simulink model "MPC_MG secondary"  (R2021b)
settings: Solver=ode23tb  StartTime=0.0  StopTime=5  RelTol=1e-3
model workspace (MAT data in the model file):
  Ts : Simulink.Parameter (value not decoded)
  secondary_on : Simulink.Parameter (value not decoded)
values from neighbouring files (symbols this model uses):
  a12 = 0    [Four_DG_MG_PrimaryOnlyScript.m]    (also in MPC_MG_script_raw_dmpc.m; MPC_MG_secondary_script.m)
  a14 = 0    [Four_DG_MG_PrimaryOnlyScript.m]    (also in MPC_MG_script_raw_dmpc.m; MPC_MG_secondary_script.m)
  a21 = 1    [Four_DG_MG_PrimaryOnlyScript.m]    (also in MPC_MG_script_raw_dmpc.m; MPC_MG_secondary_script.m)
  a23 = 0    [Four_DG_MG_PrimaryOnlyScript.m]    (also in MPC_MG_script_raw_dmpc.m; MPC_MG_secondary_script.m)
  a32 = 1    [Four_DG_MG_PrimaryOnlyScript.m]    (also in MPC_MG_script_raw_dmpc.m; MPC_MG_secondary_script.m)
  a34 = 0    [Four_DG_MG_PrimaryOnlyScript.m]    (also in MPC_MG_script_raw_dmpc.m; MPC_MG_secondary_script.m)
  a41 = 1    [Four_DG_MG_PrimaryOnlyScript.m]    (also in MPC_MG_script_raw_dmpc.m; MPC_MG_secondary_script.m)
  a43 = 0    [Four_DG_MG_PrimaryOnlyScript.m]    (also in MPC_MG_script_raw_dmpc.m; MPC_MG_secondary_script.m)
  b1v = 1    [Four_DG_MG_PrimaryOnlyScript.m]    (also in MPC_MG_script_raw_dmpc.m; MPC_MG_secondary_script.m; MPG_MG_July.m; MPG_MG_freq_script.m)
  b1w = 1    [Four_DG_MG_PrimaryOnlyScript.m]    (also in MPC_MG_script_raw_dmpc.m; MPC_MG_secondary_script.m; MPG_MG_July.m; MPG_MG_freq_script.m)
  b2v = 0    [Four_DG_MG_PrimaryOnlyScript.m]    (also in MPC_MG_script_raw_dmpc.m; MPC_MG_secondary_script.m; MPG_MG_July.m; MPG_MG_freq_script.m)
  b2w = 0    [Four_DG_MG_PrimaryOnlyScript.m]    (also in MPC_MG_script_raw_dmpc.m; MPC_MG_secondary_script.m; MPG_MG_July.m; MPG_MG_freq_script.m)
  b3v = 0    [Four_DG_MG_PrimaryOnlyScript.m]    (also in MPC_MG_script_raw_dmpc.m; MPC_MG_secondary_script.m; MPG_MG_July.m; MPG_MG_freq_script.m)
  b3w = 0    [Four_DG_MG_PrimaryOnlyScript.m]    (also in MPC_MG_script_raw_dmpc.m; MPC_MG_secondary_script.m; MPG_MG_July.m; MPG_MG_freq_script.m)
  b4v = 0    [Four_DG_MG_PrimaryOnlyScript.m]    (also in MPC_MG_script_raw_dmpc.m; MPC_MG_secondary_script.m; MPG_MG_July.m; MPG_MG_freq_script.m)
  b4w = 0    [Four_DG_MG_PrimaryOnlyScript.m]    (also in MPC_MG_script_raw_dmpc.m; MPC_MG_secondary_script.m; MPG_MG_July.m; MPG_MG_freq_script.m)
  C_f = 50e-6    (= 5e-05)    [Four_DG_MG_PrimaryOnlyScript.m]    (also in MPC_MG_script.m; MPC_MG_script_raw_dmpc.m; MPC_MG_secondary_script.m; MPG_MG_July.m)
  cf = 60    [Four_DG_MG_PrimaryOnlyScript.m]    (also in MPC_MG_script_raw_dmpc.m = 40; MPC_MG_secondary_script.m = 40; MPG_MG_July.m = 100; MPG_MG_freq_script.m = 100)
  cv = 60    [Four_DG_MG_PrimaryOnlyScript.m]    (also in MPC_MG_script_raw_dmpc.m = 40; MPC_MG_secondary_script.m = 40; MPG_MG_July.m = 100; MPG_MG_freq_script.m = 100)
  f_c = 5000    [Four_DG_MG_PrimaryOnlyScript.m]    (also in MPC_MG_script.m = 40000; MPC_MG_script_raw_dmpc.m = 40000; MPC_MG_secondary_script.m = 40000; MPG_MG_July.m = 50000)
  kL = 1e-5    (= 1e-05)    [Four_DG_MG_PrimaryOnlyScript.m]    (also in MPC_MG_script.m = 1e-08; MPC_MG_script_raw_dmpc.m = 1e-08; MPC_MG_secondary_script.m = 1e-07; MPG_MG_July.m = 1e-07)
  L_f = 1.35e-3    (= 0.00135)    [Four_DG_MG_PrimaryOnlyScript.m]    (also in MPC_MG_script.m; MPC_MG_script_raw_dmpc.m; MPC_MG_secondary_script.m; MPG_MG_July.m)
  L_in1 = 0.35e-3    (= 0.00035)    [Four_DG_MG_PrimaryOnlyScript.m]    (also in MPC_MG_script.m; MPC_MG_script_raw_dmpc.m; MPC_MG_secondary_script.m; MPG_MG_July.m)
  L_in2 = 0.35e-3    (= 0.00035)    [Four_DG_MG_PrimaryOnlyScript.m]    (also in MPC_MG_script.m; MPC_MG_script_raw_dmpc.m; MPC_MG_secondary_script.m; MPG_MG_July.m)
  L_in3 = 0.35e-3    (= 0.00035)    [Four_DG_MG_PrimaryOnlyScript.m]    (also in MPC_MG_script.m; MPC_MG_script_raw_dmpc.m; MPC_MG_secondary_script.m; MPG_MG_July.m)
  L_in4 = 0.35e-3    (= 0.00035)    [Four_DG_MG_PrimaryOnlyScript.m]    (also in MPC_MG_script.m; MPC_MG_script_raw_dmpc.m; MPC_MG_secondary_script.m; MPG_MG_July.m)
  LD_ref1 = 800e-6    (= 0.0008)    [Four_DG_MG_PrimaryOnlyScript.m]    (also in MPC_MG_script.m = 0.0003; MPC_MG_script_raw_dmpc.m = 0.0003; MPC_MG_secondary_script.m = 0.0001; MPG_MG_July.m = 0.0004)
  lo_co = 0.2    [Four_DG_MG_PrimaryOnlyScript.m]    (also in MPC_MG_script.m = 0.05; MPC_MG_script_raw_dmpc.m; MPC_MG_secondary_script.m = 0.08; MPG_MG_July.m = 0.15)
  m_p1 = 9.4e-5/droopDivide    (= 9.4e-05)    [Four_DG_MG_PrimaryOnlyScript.m]    (also in MPC_MG_script.m; MPC_MG_script_raw_dmpc.m; MPC_MG_secondary_script.m; MPG_MG_July.m)
  m_p2 = 9.4e-5/droopDivide    (= 9.4e-05)    [Four_DG_MG_PrimaryOnlyScript.m]    (also in MPC_MG_script.m; MPC_MG_script_raw_dmpc.m; MPC_MG_secondary_script.m; MPG_MG_July.m)
  m_p3 = 12.5e-5/droopDivide    (= 0.000125)    [Four_DG_MG_PrimaryOnlyScript.m]    (also in MPC_MG_script.m; MPC_MG_script_raw_dmpc.m; MPC_MG_secondary_script.m; MPG_MG_July.m)
  m_p4 = 12.5e-5/droopDivide    (= 0.000125)    [Four_DG_MG_PrimaryOnlyScript.m]    (also in MPC_MG_script.m; MPC_MG_script_raw_dmpc.m; MPC_MG_secondary_script.m; MPG_MG_July.m)
  n_q1 = 1.3e-3/droopDivide2    (= 0.00013)    [Four_DG_MG_PrimaryOnlyScript.m]    (also in MPC_MG_script.m; MPC_MG_script_raw_dmpc.m; MPC_MG_secondary_script.m; MPG_MG_July.m)
  n_q2 = 1.3e-3/droopDivide2    (= 0.00013)    [Four_DG_MG_PrimaryOnlyScript.m]    (also in MPC_MG_script.m; MPC_MG_script_raw_dmpc.m; MPC_MG_secondary_script.m; MPG_MG_July.m)
  n_q3 = 1.5e-3/droopDivide2    (= 0.00015)    [Four_DG_MG_PrimaryOnlyScript.m]    (also in MPC_MG_script.m; MPC_MG_script_raw_dmpc.m; MPC_MG_secondary_script.m; MPG_MG_July.m)
  n_q4 = 1.5e-3/droopDivide2    (= 0.00015)    [Four_DG_MG_PrimaryOnlyScript.m]    (also in MPC_MG_script.m; MPC_MG_script_raw_dmpc.m; MPC_MG_secondary_script.m; MPG_MG_July.m)
  R_f = 0.1    [Four_DG_MG_PrimaryOnlyScript.m]    (also in MPC_MG_script.m; MPC_MG_script_raw_dmpc.m; MPC_MG_secondary_script.m; MPG_MG_July.m)
  R_in1 = 0.03    [Four_DG_MG_PrimaryOnlyScript.m]    (also in MPC_MG_script.m; MPC_MG_script_raw_dmpc.m; MPC_MG_secondary_script.m; MPG_MG_July.m)
  R_in2 = 0.03    [Four_DG_MG_PrimaryOnlyScript.m]    (also in MPC_MG_script.m; MPC_MG_script_raw_dmpc.m; MPC_MG_secondary_script.m; MPG_MG_July.m)
  R_in3 = 0.03    [Four_DG_MG_PrimaryOnlyScript.m]    (also in MPC_MG_script.m; MPC_MG_script_raw_dmpc.m; MPC_MG_secondary_script.m; MPG_MG_July.m)
  R_in4 = 0.03    [Four_DG_MG_PrimaryOnlyScript.m]    (also in MPC_MG_script.m; MPC_MG_script_raw_dmpc.m; MPC_MG_secondary_script.m; MPG_MG_July.m)
  time_thresh = 0.6    [Four_DG_MG_PrimaryOnlyScript.m]    (also in MPC_MG_script_raw_dmpc.m = 1.5; MPC_MG_secondary_script.m = 2; MPG_MG_July.m = 0.5; MPG_MG_freq_script.m = 0.5)
  Ts = 10e-6    (= 1e-05)    [Four_DG_MG_PrimaryOnlyScript.m]    (also in MPC_MG_script.m; MPC_MG_script_raw_dmpc.m; MPC_MG_secondary_script.m; MPG_MG_July.m)
  V_nom = 220*sqrt(2)    [Four_DG_MG_PrimaryOnlyScript.m]    (also in MPC_MG_script.m; MPC_MG_script_raw_dmpc.m; MPC_MG_secondary_script.m; MPG_MG_July.m)
  Vdc = 600    [Four_DG_MG_PrimaryOnlyScript.m]    (also in MPC_MG_script.m; MPC_MG_script_raw_dmpc.m; MPC_MG_secondary_script.m; MPG_MG_July.m)
  w_c_high = 2*pi*50    (= 314.159265359)    [Four_DG_MG_PrimaryOnlyScript.m]    (also in MPC_MG_script.m; MPC_MG_script_raw_dmpc.m; MPC_MG_secondary_script.m; MPG_MG_July.m)
  w_nom = 2*pi*50    (= 314.159265359)    [Four_DG_MG_PrimaryOnlyScript.m]    (also in MPC_MG_script.m; MPC_MG_script_raw_dmpc.m; MPC_MG_secondary_script.m; MPG_MG_July.m)
undefined symbols (not defined in the file or in its folder): i
libraries: spsThreePhaseSeriesRLCBranchLib x18, spsThreePhaseVIMeasurementLib x12, spsabctodq0Lib x12, eeGeneralControl x10, dspswit3 x5, powerlib x5, spsPMUPLLBasedPositiveSequenceLib x4, spsDCVoltageSourceLib x4, spsSeriesRLCBranchLib x4, spsTwoLevelConverterLib x4, spsThreePhaseSeriesRLCLoadLib x3, powerlib_meascontrol x3
(part 3 of 3)

== system MPC_MG secondary/Voltage Source Inverter 4/3to2 1 ==
  "Vabc_o " : Inport
  Add : Sum  Inputs=+++
  Constant : Constant  Value=exp(i*2*pi/3)
  Constant1 : Constant  Value=2/3
  Demux : Demux  Outputs=3
  Math Function : Math  Operator=square  SignedPower=on  SaturateOnIntegerOverflow=on
  Product : Product  RndMeth=Zero
  Product1 : Product  RndMeth=Zero
  Product2 : Product  RndMeth=Zero
  Vo : Outport  VectorParamsAs1DForOutWhenUnconnected=off
  wires:
  Add/1 -> Product/1
  Demux/1 -> Add/1
  Constant1/1 -> Product/2
  Product1/1 -> Add/2
  Constant/1 -> Product1/1, Math Function/1
  Demux/2 -> Product1/2
  Math Function/1 -> Product2/1
  Demux/3 -> Product2/2
  Product2/1 -> Add/3
  Product/1 -> Vo/1
  "Vabc_o "/1 -> Demux/1

== system MPC_MG secondary/Voltage Source Inverter 4/3to2 2 ==
  "Iabc_o " : Inport
  Add : Sum  Inputs=+++
  Constant : Constant  Value=exp(i*2*pi/3)
  Constant1 : Constant  Value=2/3
  Demux : Demux  Outputs=3
  Math Function : Math  Operator=square  SignedPower=on  SaturateOnIntegerOverflow=on
  Product : Product  RndMeth=Zero
  Product1 : Product  RndMeth=Zero
  Product2 : Product  RndMeth=Zero
  Il : Outport  VectorParamsAs1DForOutWhenUnconnected=off
  wires:
  Add/1 -> Product/1
  Demux/1 -> Add/1
  Constant1/1 -> Product/2
  Product1/1 -> Add/2
  Constant/1 -> Product1/1, Math Function/1
  Demux/2 -> Product1/2
  Math Function/1 -> Product2/1
  Demux/3 -> Product2/2
  Product2/1 -> Add/3
  Product/1 -> Il/1
  "Iabc_o "/1 -> Demux/1

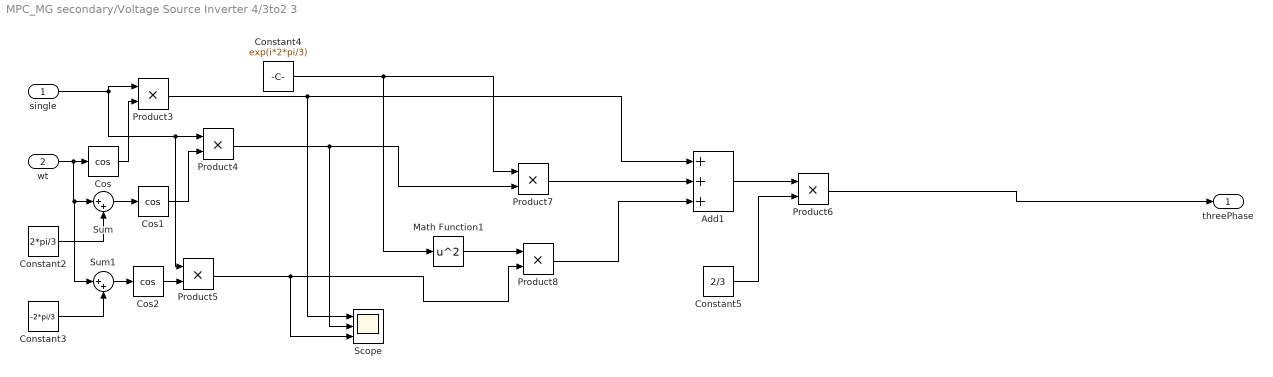
== system MPC_MG secondary/Voltage Source Inverter 4/3to2 3 ==
  "single " : Inport
  "wt " : Inport  Port=2
  Add1 : Sum  Inputs=+++
  Constant2 : Constant  Value=2*pi/3
  Constant3 : Constant  Value=-2*pi/3
  Constant4 : Constant  Value=exp(i*2*pi/3)
  Constant5 : Constant  Value=2/3
  Cos : Trigonometry  Operator=cos
  Cos1 : Trigonometry  Operator=cos
  Cos2 : Trigonometry  Operator=cos
  Math Function1 : Math  Operator=square  SignedPower=on  SaturateOnIntegerOverflow=on
  Product{3..8} (6 alike) : Product  RndMeth=Zero
  Scope : Scope  NumInputPorts=3
  Sum : Sum  Inputs=|++
  Sum1 : Sum  Inputs=|++
  threePhase : Outport  VectorParamsAs1DForOutWhenUnconnected=off
  wires:
  "single "/1 -> Product5/1, Product4/1, Product3/1
  Cos/1 -> Product3/2
  Constant2/1 -> Sum/2
  Sum/1 -> Cos1/1
  Cos1/1 -> Product4/2
  "wt "/1 -> Sum1/1, Sum/1, Cos/1
  Constant3/1 -> Sum1/2
  Sum1/1 -> Cos2/1
  Cos2/1 -> Product5/2
  Constant4/1 -> Product7/1, Math Function1/1
  Product7/1 -> Add1/2
  Add1/1 -> Product6/1
  Product8/1 -> Add1/3
  Product5/1 -> Scope/3, Product8/2
  Product6/1 -> threePhase/1
  Product3/1 -> Scope/1, Add1/1
  Constant5/1 -> Product6/2
  Product4/1 -> Scope/2, Product7/2
  Math Function1/1 -> Product8/1

== system MPC_MG secondary/Voltage Source Inverter 4/Droop for secondary control2 ==
  P : Inport
  w_nom : Inport  Port=2
  V_nom : Inport  Port=3
  Q : Inport  Port=4
  Gain4 : Gain  Gain=n_q
  Gain5 : Gain  Gain=m_p
  Integrator : Integrator  WrapState=on  WrappedStateUpperValue=2*pi  WrappedStateLowerValue=0
  Sum1 : Sum  Inputs=|+-
  Sum2 : Sum  Inputs=|+-
  Vref : Outport
  wt : Outport  Port=2
  wo : Outport  Port=3
  wires:
  P/1 -> Gain5/1
  w_nom/1 -> Sum2/1
  Gain5/1 -> Sum2/2
  Sum2/1 -> wo/1, Integrator/1  "w"
  Integrator/1 -> wt/1
  V_nom/1 -> Sum1/1  "Vod_s"
  Gain4/1 -> Sum1/2
  Q/1 -> Gain4/1
  Sum1/1 -> Vref/1  "Vod_s"

== system MPC_MG secondary/Voltage Source Inverter 4/Low-pass filter ==
  p_hat : Inport
  q_hat : Inport  Port=2
  Low-Pass Filter (Discrete or Continuous) : eeGeneralControl/Low-Pass Filter (Discrete or Continuous)  K=1  T=lo_co  B=inf  A=-inf  init_option=Inherited from block input  x0=0  Ts=-1
  Low-Pass Filter (Discrete or Continuous)1 : eeGeneralControl/Low-Pass Filter (Discrete or Continuous)  K=1  T=lo_co  B=inf  A=-inf  init_option=Inherited from block input  x0=0  Ts=-1
  P : Outport
  Q : Outport  Port=2
  wires:
  q_hat/1 -> Low-Pass Filter (Discrete or Continuous)1/1
  Low-Pass Filter (Discrete or Continuous)1/1 -> Q/1  "Q"
  Low-Pass Filter (Discrete or Continuous)/1 -> P/1  "P"
  p_hat/1 -> Low-Pass Filter (Discrete or Continuous)/1

== system MPC_MG secondary/Voltage Source Inverter 4/PQ calculator ==
  Vod : Inport
  Voq : Inport  Port=2
  Iod : Inport  Port=3
  Ioq : Inport  Port=4
  Product{,1..3} (4 alike) : Product
  Sum10 : Sum  Inputs=|++
  Sum11 : Sum  Inputs=|+-
  p_hat : Outport
  q_hat : Outport  Port=2
  wires:
  Product3/1 -> Sum11/2
  Product1/1 -> Sum10/2
  Voq/1 -> Product3/1, Product1/1
  Iod/1 -> Product/2, Product3/2
  Product2/1 -> Sum11/1
  Ioq/1 -> Product1/2, Product2/2
  Product/1 -> Sum10/1
  Vod/1 -> Product/1, Product2/1
  Sum11/1 -> q_hat/1  "q_hat"
  Sum10/1 -> p_hat/1  "p_hat"

== system MPC_MG secondary/Voltage Source Inverter 4/dq converter ==
  Vodq : Inport
  Iodq : Inport  Port=2
  Ildq : Inport  Port=3
  wo : Inport  Port=4
  Demux : Demux  Outputs=2
  Demux1 : Demux  Outputs=2
  Demux4 : Demux  Outputs=2
  Selector1 : Selector  InputPortWidth=3  IndexOptions=Index vector (dialog)  Indices=[1 2]  OutputSizes=1
  Selector2 : Selector  InputPortWidth=3  IndexOptions=Index vector (dialog)  Indices=[1 2]  OutputSizes=1
  Selector3 : Selector  InputPortWidth=3  IndexOptions=Index vector (dialog)  Indices=[1 2]  OutputSizes=1
  abc to dq0 : spsabctodq0Lib/abc to dq0  Alignment=90 degrees behind phase A axis
  abc to dq1 : spsabctodq0Lib/abc to dq0  Alignment=90 degrees behind phase A axis
  abc to dq2 : spsabctodq0Lib/abc to dq0  Alignment=90 degrees behind phase A axis
  Vod : Outport
  Voq : Outport  Port=2
  Iod : Outport  Port=3
  Ioq : Outport  Port=4
  Ild : Outport  Port=5
  Ilq : Outport  Port=6
  tag scope: Vod4=global
  wires:
  Vodq/1 -> abc to dq0/1
  Demux/1 -> [Vod4], Vod/1  "Vod"
  Demux1/1 -> Iod/1  "Iod"
  Selector3/1 -> Demux4/1
  Demux/2 -> Voq/1  "Voq"
  Selector1/1 -> Demux/1
  abc to dq2/1 -> Selector2/1
  abc to dq1/1 -> Selector3/1
  wo/1 -> abc to dq0/2, abc to dq2/2, abc to dq1/2
  Demux1/2 -> Ioq/1  "Ioq"
  Demux4/1 -> Ild/1  "Ild"
  abc to dq0/1 -> Selector1/1
  Selector2/1 -> Demux1/1
  Iodq/1 -> abc to dq2/1
  Ildq/1 -> abc to dq1/1
  Demux4/2 -> Ilq/1  "Ilq"

== system MPC_MG secondary/Voltage Source Inverter 4/remap ==
  In1 : Inport
  Demux : Demux  Outputs=6
  Mux : Mux  Inputs=6
  Out1 : Outport
  wires:
  Demux/5 -> Mux/4
  Demux/3 -> Mux/5
  Demux/2 -> Mux/3
  Demux/4 -> Mux/2
  In1/1 -> Demux/1
  Demux/1 -> Mux/1
  Demux/6 -> Mux/6
  Mux/1 -> Out1/1

== system MPC_MG secondary/Voltage Source Inverter 5/3to2 1 ==
  "Vabc_o " : Inport
  Add : Sum  Inputs=+++
  Constant : Constant  Value=exp(i*2*pi/3)
  Constant1 : Constant  Value=2/3
  Demux : Demux  Outputs=3
  Math Function : Math  Operator=square  SignedPower=on  SaturateOnIntegerOverflow=on
  Product : Product  RndMeth=Zero
  Product1 : Product  RndMeth=Zero
  Product2 : Product  RndMeth=Zero
  Vo : Outport  VectorParamsAs1DForOutWhenUnconnected=off
  wires:
  Add/1 -> Product/1
  Demux/1 -> Add/1
  Constant1/1 -> Product/2
  Product1/1 -> Add/2
  Constant/1 -> Product1/1, Math Function/1
  Demux/2 -> Product1/2
  Math Function/1 -> Product2/1
  Demux/3 -> Product2/2
  Product2/1 -> Add/3
  Product/1 -> Vo/1
  "Vabc_o "/1 -> Demux/1

== system MPC_MG secondary/Voltage Source Inverter 5/3to2 2 ==
  "Iabc_o " : Inport
  Add : Sum  Inputs=+++
  Constant : Constant  Value=exp(i*2*pi/3)
  Constant1 : Constant  Value=2/3
  Demux : Demux  Outputs=3
  Math Function : Math  Operator=square  SignedPower=on  SaturateOnIntegerOverflow=on
  Product : Product  RndMeth=Zero
  Product1 : Product  RndMeth=Zero
  Product2 : Product  RndMeth=Zero
  Il : Outport  VectorParamsAs1DForOutWhenUnconnected=off
  wires:
  Add/1 -> Product/1
  Demux/1 -> Add/1
  Constant1/1 -> Product/2
  Product1/1 -> Add/2
  Constant/1 -> Product1/1, Math Function/1
  Demux/2 -> Product1/2
  Math Function/1 -> Product2/1
  Demux/3 -> Product2/2
  Product2/1 -> Add/3
  Product/1 -> Il/1
  "Iabc_o "/1 -> Demux/1

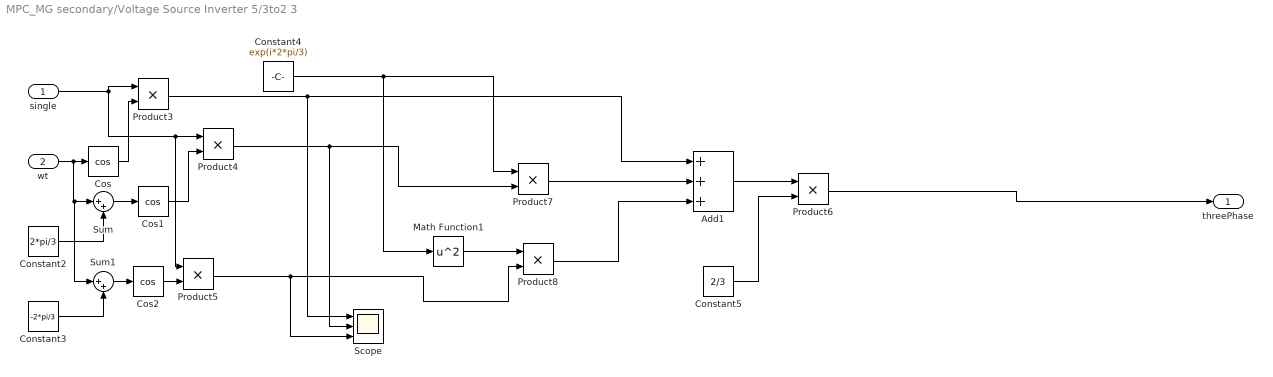
== system MPC_MG secondary/Voltage Source Inverter 5/3to2 3 ==
  "single " : Inport
  "wt " : Inport  Port=2
  Add1 : Sum  Inputs=+++
  Constant2 : Constant  Value=2*pi/3
  Constant3 : Constant  Value=-2*pi/3
  Constant4 : Constant  Value=exp(i*2*pi/3)
  Constant5 : Constant  Value=2/3
  Cos : Trigonometry  Operator=cos
  Cos1 : Trigonometry  Operator=cos
  Cos2 : Trigonometry  Operator=cos
  Math Function1 : Math  Operator=square  SignedPower=on  SaturateOnIntegerOverflow=on
  Product{3..8} (6 alike) : Product  RndMeth=Zero
  Scope : Scope  NumInputPorts=3
  Sum : Sum  Inputs=|++
  Sum1 : Sum  Inputs=|++
  threePhase : Outport  VectorParamsAs1DForOutWhenUnconnected=off
  wires:
  "single "/1 -> Product5/1, Product4/1, Product3/1
  Cos/1 -> Product3/2
  Constant2/1 -> Sum/2
  Sum/1 -> Cos1/1
  Cos1/1 -> Product4/2
  "wt "/1 -> Sum1/1, Sum/1, Cos/1
  Constant3/1 -> Sum1/2
  Sum1/1 -> Cos2/1
  Cos2/1 -> Product5/2
  Constant4/1 -> Product7/1, Math Function1/1
  Product7/1 -> Add1/2
  Add1/1 -> Product6/1
  Product8/1 -> Add1/3
  Product5/1 -> Scope/3, Product8/2
  Product6/1 -> threePhase/1
  Product3/1 -> Scope/1, Add1/1
  Constant5/1 -> Product6/2
  Product4/1 -> Scope/2, Product7/2
  Math Function1/1 -> Product8/1

== system MPC_MG secondary/Voltage Source Inverter 5/Droop for secondary control2 ==
  P : Inport
  w_nom : Inport  Port=2
  V_nom : Inport  Port=3
  Q : Inport  Port=4
  Gain4 : Gain  Gain=n_q
  Gain5 : Gain  Gain=m_p
  Integrator : Integrator  WrapState=on  WrappedStateUpperValue=2*pi  WrappedStateLowerValue=0
  Sum1 : Sum  Inputs=|+-
  Sum2 : Sum  Inputs=|+-
  Vref : Outport
  wt : Outport  Port=2
  wo : Outport  Port=3
  wires:
  P/1 -> Gain5/1
  w_nom/1 -> Sum2/1
  Gain5/1 -> Sum2/2
  Sum2/1 -> wo/1, Integrator/1  "w"
  Integrator/1 -> wt/1
  V_nom/1 -> Sum1/1  "Vod_s"
  Gain4/1 -> Sum1/2
  Q/1 -> Gain4/1
  Sum1/1 -> Vref/1  "Vod_s"

== system MPC_MG secondary/Voltage Source Inverter 5/Low-pass filter ==
  p_hat : Inport
  q_hat : Inport  Port=2
  Low-Pass Filter (Discrete or Continuous) : eeGeneralControl/Low-Pass Filter (Discrete or Continuous)  K=1  T=lo_co  B=inf  A=-inf  init_option=Inherited from block input  x0=0  Ts=-1
  Low-Pass Filter (Discrete or Continuous)1 : eeGeneralControl/Low-Pass Filter (Discrete or Continuous)  K=1  T=lo_co  B=inf  A=-inf  init_option=Inherited from block input  x0=0  Ts=-1
  P : Outport
  Q : Outport  Port=2
  wires:
  q_hat/1 -> Low-Pass Filter (Discrete or Continuous)1/1
  Low-Pass Filter (Discrete or Continuous)1/1 -> Q/1  "Q"
  Low-Pass Filter (Discrete or Continuous)/1 -> P/1  "P"
  p_hat/1 -> Low-Pass Filter (Discrete or Continuous)/1

== system MPC_MG secondary/Voltage Source Inverter 5/PQ calculator ==
  Vod : Inport
  Voq : Inport  Port=2
  Iod : Inport  Port=3
  Ioq : Inport  Port=4
  Product{,1..3} (4 alike) : Product
  Sum10 : Sum  Inputs=|++
  Sum11 : Sum  Inputs=|+-
  p_hat : Outport
  q_hat : Outport  Port=2
  wires:
  Product3/1 -> Sum11/2
  Product1/1 -> Sum10/2
  Voq/1 -> Product3/1, Product1/1
  Iod/1 -> Product/2, Product3/2
  Product2/1 -> Sum11/1
  Ioq/1 -> Product1/2, Product2/2
  Product/1 -> Sum10/1
  Vod/1 -> Product/1, Product2/1
  Sum11/1 -> q_hat/1  "q_hat"
  Sum10/1 -> p_hat/1  "p_hat"

== system MPC_MG secondary/Voltage Source Inverter 5/dq converter ==
  Vodq : Inport
  Iodq : Inport  Port=2
  Ildq : Inport  Port=3
  wo : Inport  Port=4
  Demux : Demux  Outputs=2
  Demux1 : Demux  Outputs=2
  Demux4 : Demux  Outputs=2
  Selector1 : Selector  InputPortWidth=3  IndexOptions=Index vector (dialog)  Indices=[1 2]  OutputSizes=1
  Selector2 : Selector  InputPortWidth=3  IndexOptions=Index vector (dialog)  Indices=[1 2]  OutputSizes=1
  Selector3 : Selector  InputPortWidth=3  IndexOptions=Index vector (dialog)  Indices=[1 2]  OutputSizes=1
  abc to dq0 : powerlib_meascontrol/Transformations/abc to dq0  Alignment=90 degrees behind phase A axis
  abc to dq1 : powerlib_meascontrol/Transformations/abc to dq0  Alignment=90 degrees behind phase A axis
  abc to dq2 : powerlib_meascontrol/Transformations/abc to dq0  Alignment=90 degrees behind phase A axis
  Vod : Outport
  Voq : Outport  Port=2
  Iod : Outport  Port=3
  Ioq : Outport  Port=4
  Ild : Outport  Port=5
  Ilq : Outport  Port=6
  wires:
  Vodq/1 -> abc to dq0/1
  Demux/1 -> Vod/1  "Vod"
  Demux1/1 -> Iod/1  "Iod"
  Selector3/1 -> Demux4/1
  Demux/2 -> Voq/1  "Voq"
  Selector1/1 -> Demux/1
  abc to dq2/1 -> Selector2/1
  abc to dq1/1 -> Selector3/1
  wo/1 -> abc to dq0/2, abc to dq2/2, abc to dq1/2
  Demux1/2 -> Ioq/1  "Ioq"
  Demux4/1 -> Ild/1  "Ild"
  abc to dq0/1 -> Selector1/1
  Selector2/1 -> Demux1/1
  Iodq/1 -> abc to dq2/1
  Ildq/1 -> abc to dq1/1
  Demux4/2 -> Ilq/1  "Ilq"

== system MPC_MG secondary/Voltage Source Inverter 5/remap ==
  In1 : Inport
  Demux : Demux  Outputs=6
  Mux : Mux  Inputs=6
  Out1 : Outport
  wires:
  Demux/5 -> Mux/4
  Demux/3 -> Mux/5
  Demux/2 -> Mux/3
  Demux/4 -> Mux/2
  In1/1 -> Demux/1
  Demux/1 -> Mux/1
  Demux/6 -> Mux/6
  Mux/1 -> Out1/1

== matlab function MPC_MG secondary/Voltage Source Inverter 5/Model Predictive Control  ==
  settings: updateMethod=DISCRETE  sampleTime=Ts
  data: S_opt output; Sopt output size=[1 6]; Vc input; i_filter input; vref input; Vi_opt output; Vdc parameter double size=1; modT parameter size=1; Cfilter parameter size=1; Lfilter parameter size=1
function [S_opt, Sopt, Vi_opt] = MPC(Vc, i_filter,vref,Vdc,modT,Cfilter,Lfilter)

    % In order to call "cont2dis" function
    coder.extrinsic('cont2dis');
    persistent Aq Bq Bdq Vc1 if1 Vc_old if_old x_opt g f_window f_window2 fil fil2

    % Initialize variables and get the parameters of the Discrete model based on Ts
    if isempty(x_opt), x_opt = 1; end
    if isempty(Vc1), Vc1 = 0 + 1j*0; end
    if isempty(Vc_old), Vc_old = 0 + 1j*0; end
    if isempty(if_old), if_old = 0 + 1j*0; end
    if isempty(if1), if1 = 0 + 1j*0; end
    if isempty(f_window), f_window = zeros(1,51); end
    if isempty(f_window2), f_window2 = zeros(1,51); end

    if isempty(Aq) && isempty(Bq) && isempty(Bdq)
        Aq = zeros(2);     Bq = zeros(2,1);     Bdq = zeros(2,1);
        % Call "cont2dis" function
        [Aq, Bq, Bdq] = cont2dis(modT,Lfilter,Cfilter); 
    end
    
    % Intialize the cost function
    g_opt = inf;
    
    % To generate the switching states matrix
    states = [1 0 0;
              0 0 0  
              1 1 0
              0 1 0
              0 1 1
              0 0 1
              1 0 1
              1 1 1];
    a = exp(1j*(2*pi/3));
    %notch filter
    fil = fir1(2,[0.1225 0.1275],'DC-0');
    fil2 = fir1(2,[0.1225 0.1275],'DC-0');
    
    % Read current measurements at sampling instant k
    ifk = i_filter;
    Vck = Vc;
    % Equation of io(k-1) = if(k-1)-(c/Ts)(vc(k)-vc(k-1)).
    io = if_old - (Cfilter/modT)*(Vck - Vc_old); 
    
    % Store the measured current for the next iteration
    if_old = ifk;
    Vc_old = Vck;
    % FOR loop to find the best switch in the next instant and its corresponding V(i)
    for k = 1:8
        s = states(k,:);
        sw = (2/3)*(s(1)+a*s(2)+a^2*s(3));
        Vi = Vdc*sw;

        % Output Voltage Prediction at instant k+1
        if1 = Aq(1,1)*ifk + Aq(1,2)*Vck + Bq(1)*Vi + Bdq(1)*io; 
        Vc1 = Aq(2,1)*ifk + Aq(2,2)*Vck + Bq(2)*Vi + Bdq(2)*io; 
        Nc = sum(abs(states(k,:)-states(x_opt,:)))^2;    
        gf = filter(fil, 1, f_window);
        gf2 = filter(fil2, 1, f_window2);
        g1 = (real(if1)-real(io)+Cfilter*2*pi*50*imag(vref))^2 + (imag(if1)-imag(io)+Cfilter*2*pi*50*real(vref))^2;
        g = (real(vref)-real(Vc1))^2+(imag(vref)-imag(Vc1))^2 + 0.1*g1 + 3*Nc + 3*gf(1) + 3*gf2(1);
        if (g < g_opt)
            x_opt = k;
            g_opt = g;
            f_window = [sqrt((real(vref)-real(Vc1))^2+(imag(vref)-imag(Vc1))^2), f_window(1:(length(f_window)-1))];
            f_window2 = [g, f_window2(1:(length(f_window2)-1))];
        end
             
    end
    
    % Output switching states and its voltage vector. 
    Vi_opt = x_opt; 
    S_opt = states(x_opt,:);
    d_opt = not(S_opt);
    Sopt = [S_opt,d_opt];     

end

== matlab function MPC_MG secondary/Voltage Source Inverter 2/Model Predictive Control  ==
  settings: updateMethod=DISCRETE  sampleTime=Ts
  data: S_opt output; Sopt output size=[1 6]; Vc input; i_filter input; vref input; Vi_opt output; Vdc parameter double size=1; modT parameter size=1; Cfilter parameter size=1; Lfilter parameter size=1
function [S_opt, Sopt, Vi_opt] = MPC(Vc, i_filter,vref,Vdc,modT,Cfilter,Lfilter)

    % In order to call "cont2dis" function
    coder.extrinsic('cont2dis');
    persistent Aq Bq Bdq Vc1 if1 Vc_old if_old x_opt g f_window f_window2 fil fil2

    % Initialize variables and get the parameters of the Discrete model based on Ts
    if isempty(x_opt), x_opt = 1; end
    if isempty(Vc1), Vc1 = 0 + 1j*0; end
    if isempty(Vc_old), Vc_old = 0 + 1j*0; end
    if isempty(if_old), if_old = 0 + 1j*0; end
    if isempty(if1), if1 = 0 + 1j*0; end
    if isempty(f_window), f_window = zeros(1,51); end
    if isempty(f_window2), f_window2 = zeros(1,51); end

    if isempty(Aq) && isempty(Bq) && isempty(Bdq)
        Aq = zeros(2);     Bq = zeros(2,1);     Bdq = zeros(2,1);
        % Call "cont2dis" function
        [Aq, Bq, Bdq] = cont2dis(modT,Lfilter,Cfilter); 
    end
    
    % Intialize the cost function
    g_opt = inf;
    
    % To generate the switching states matrix
    states = [1 0 0;
              0 0 0  
              1 1 0
              0 1 0
              0 1 1
              0 0 1
              1 0 1
              1 1 1];
    a = exp(1j*(2*pi/3));
    %notch filter
    fil = fir1(2,[0.1225 0.1275],'DC-0');
    fil2 = fir1(2,[0.1225 0.1275],'DC-0');
    
    % Read current measurements at sampling instant k
    ifk = i_filter;
    Vck = Vc;
    % Equation of io(k-1) = if(k-1)-(c/Ts)(vc(k)-vc(k-1)).
    io = if_old - (Cfilter/modT)*(Vck - Vc_old); 
    
    % Store the measured current for the next iteration
    if_old = ifk;
    Vc_old = Vck;
    % FOR loop to find the best switch in the next instant and its corresponding V(i)
    for k = 1:8
        s = states(k,:);
        sw = (2/3)*(s(1)+a*s(2)+a^2*s(3));
        Vi = Vdc*sw;

        % Output Voltage Prediction at instant k+1
        if1 = Aq(1,1)*ifk + Aq(1,2)*Vck + Bq(1)*Vi + Bdq(1)*io; 
        Vc1 = Aq(2,1)*ifk + Aq(2,2)*Vck + Bq(2)*Vi + Bdq(2)*io; 
        Nc = sum(abs(states(k,:)-states(x_opt,:)))^2;    
        gf = filter(fil, 1, f_window);
        gf2 = filter(fil2, 1, f_window2);
        g1 = (real(if1)-real(io)+Cfilter*2*pi*50*imag(vref))^2 + (imag(if1)-imag(io)+Cfilter*2*pi*50*real(vref))^2;
        g = (real(vref)-real(Vc1))^2+(imag(vref)-imag(Vc1))^2 + 0.1*g1 + 3*Nc + 3*gf(1) + 3*gf2(1);
        if (g < g_opt)
            x_opt = k;
            g_opt = g;
            f_window = [sqrt((real(vref)-real(Vc1))^2+(imag(vref)-imag(Vc1))^2), f_window(1:(length(f_window)-1))];
            f_window2 = [g, f_window2(1:(length(f_window2)-1))];
        end
             
    end
    
    % Output switching states and its voltage vector. 
    Vi_opt = x_opt; 
    S_opt = states(x_opt,:);
    d_opt = not(S_opt);
    Sopt = [S_opt,d_opt];     

end

== matlab function MPC_MG secondary/Voltage Source Inverter 1/Model Predictive Control  ==
  settings: updateMethod=DISCRETE  sampleTime=Ts
  data: S_opt output; Sopt output size=[1 6]; Vc input; i_filter input; vref input; Vi_opt output; Vdc parameter double size=1; modT parameter size=1; Cfilter parameter size=1; Lfilter parameter size=1
function [S_opt, Sopt, Vi_opt] = MPC(Vc, i_filter,vref,Vdc,modT,Cfilter,Lfilter)

    % In order to call "cont2dis" function
    coder.extrinsic('cont2dis');
    persistent Aq Bq Bdq Vc1 if1 Vc_old if_old x_opt g f_window f_window2 fil fil2

    % Initialize variables and get the parameters of the Discrete model based on Ts
    if isempty(x_opt), x_opt = 1; end
    if isempty(Vc1), Vc1 = 0 + 1j*0; end
    if isempty(Vc_old), Vc_old = 0 + 1j*0; end
    if isempty(if_old), if_old = 0 + 1j*0; end
    if isempty(if1), if1 = 0 + 1j*0; end
    if isempty(f_window), f_window = zeros(1,51); end
    if isempty(f_window2), f_window2 = zeros(1,51); end

    if isempty(Aq) && isempty(Bq) && isempty(Bdq)
        Aq = zeros(2);     Bq = zeros(2,1);     Bdq = zeros(2,1);
        % Call "cont2dis" function
        [Aq, Bq, Bdq] = cont2dis(modT,Lfilter,Cfilter); 
    end
    
    % Intialize the cost function
    g_opt = inf;
    
    % To generate the switching states matrix
    states = [1 0 0;
              0 0 0  
              1 1 0
              0 1 0
              0 1 1
              0 0 1
              1 0 1
              1 1 1];
    a = exp(1j*(2*pi/3));
    %notch filter
    fil = fir1(2,[0.1225 0.1275],'DC-0');
    fil2 = fir1(2,[0.1225 0.1275],'DC-0');
    
    % Read current measurements at sampling instant k
    ifk = i_filter;
    Vck = Vc;
    % Equation of io(k-1) = if(k-1)-(c/Ts)(vc(k)-vc(k-1)).
    io = if_old - (Cfilter/modT)*(Vck - Vc_old); 
    
    % Store the measured current for the next iteration
    if_old = ifk;
    Vc_old = Vck;
    % FOR loop to find the best switch in the next instant and its corresponding V(i)
    for k = 1:8
        s = states(k,:);
        sw = (2/3)*(s(1)+a*s(2)+a^2*s(3));
        Vi = Vdc*sw;

        % Output Voltage Prediction at instant k+1
        if1 = Aq(1,1)*ifk + Aq(1,2)*Vck + Bq(1)*Vi + Bdq(1)*io; 
        Vc1 = Aq(2,1)*ifk + Aq(2,2)*Vck + Bq(2)*Vi + Bdq(2)*io; 
        Nc = sum(abs(states(k,:)-states(x_opt,:)))^2;    
        gf = filter(fil, 1, f_window);
        gf2 = filter(fil2, 1, f_window2);
        g1 = (real(if1)-real(io)+Cfilter*2*pi*50*imag(vref))^2 + (imag(if1)-imag(io)+Cfilter*2*pi*50*real(vref))^2;
        g = (real(vref)-real(Vc1))^2+(imag(vref)-imag(Vc1))^2 + 0.1*g1 + 3*Nc + 3*gf(1) + 3*gf2(1);
        if (g < g_opt)
            x_opt = k;
            g_opt = g;
            f_window = [sqrt((real(vref)-real(Vc1))^2+(imag(vref)-imag(Vc1))^2), f_window(1:(length(f_window)-1))];
            f_window2 = [g, f_window2(1:(length(f_window2)-1))];
        end
             
    end
    
    % Output switching states and its voltage vector. 
    Vi_opt = x_opt; 
    S_opt = states(x_opt,:);
    d_opt = not(S_opt);
    Sopt = [S_opt,d_opt];     

end

== matlab function MPC_MG secondary/Voltage Source Inverter 3/Model Predictive Control  ==
  settings: updateMethod=DISCRETE  sampleTime=Ts
  data: S_opt output; Sopt output size=[1 6]; Vc input; i_filter input; vref input; Vi_opt output; Vdc parameter double size=1; modT parameter size=1; Cfilter parameter size=1; Lfilter parameter size=1
function [S_opt, Sopt, Vi_opt] = MPC(Vc, i_filter,vref,Vdc,modT,Cfilter,Lfilter)

    % In order to call "cont2dis" function
    coder.extrinsic('cont2dis');
    persistent Aq Bq Bdq Vc1 if1 Vc_old if_old x_opt g f_window f_window2 fil fil2

    % Initialize variables and get the parameters of the Discrete model based on Ts
    if isempty(x_opt), x_opt = 1; end
    if isempty(Vc1), Vc1 = 0 + 1j*0; end
    if isempty(Vc_old), Vc_old = 0 + 1j*0; end
    if isempty(if_old), if_old = 0 + 1j*0; end
    if isempty(if1), if1 = 0 + 1j*0; end
    if isempty(f_window), f_window = zeros(1,51); end
    if isempty(f_window2), f_window2 = zeros(1,51); end

    if isempty(Aq) && isempty(Bq) && isempty(Bdq)
        Aq = zeros(2);     Bq = zeros(2,1);     Bdq = zeros(2,1);
        % Call "cont2dis" function
        [Aq, Bq, Bdq] = cont2dis(modT,Lfilter,Cfilter); 
    end
    
    % Intialize the cost function
    g_opt = inf;
    
    % To generate the switching states matrix
    states = [1 0 0;
              0 0 0  
              1 1 0
              0 1 0
              0 1 1
              0 0 1
              1 0 1
              1 1 1];
    a = exp(1j*(2*pi/3));
    %notch filter
    fil = fir1(2,[0.1225 0.1275],'DC-0');
    fil2 = fir1(2,[0.1225 0.1275],'DC-0');
    
    % Read current measurements at sampling instant k
    ifk = i_filter;
    Vck = Vc;
    % Equation of io(k-1) = if(k-1)-(c/Ts)(vc(k)-vc(k-1)).
    io = if_old - (Cfilter/modT)*(Vck - Vc_old); 
    
    % Store the measured current for the next iteration
    if_old = ifk;
    Vc_old = Vck;
    % FOR loop to find the best switch in the next instant and its corresponding V(i)
    for k = 1:8
        s = states(k,:);
        sw = (2/3)*(s(1)+a*s(2)+a^2*s(3));
        Vi = Vdc*sw;

        % Output Voltage Prediction at instant k+1
        if1 = Aq(1,1)*ifk + Aq(1,2)*Vck + Bq(1)*Vi + Bdq(1)*io; 
        Vc1 = Aq(2,1)*ifk + Aq(2,2)*Vck + Bq(2)*Vi + Bdq(2)*io; 
        Nc = sum(abs(states(k,:)-states(x_opt,:)))^2;    
        gf = filter(fil, 1, f_window);
        gf2 = filter(fil2, 1, f_window2);
        g1 = (real(if1)-real(io)+Cfilter*2*pi*50*imag(vref))^2 + (imag(if1)-imag(io)+Cfilter*2*pi*50*real(vref))^2;
        g = (real(vref)-real(Vc1))^2+(imag(vref)-imag(Vc1))^2 + 0.1*g1 + 3*Nc + 3*gf(1) + 3*gf2(1);
        if (g < g_opt)
            x_opt = k;
            g_opt = g;
            f_window = [sqrt((real(vref)-real(Vc1))^2+(imag(vref)-imag(Vc1))^2), f_window(1:(length(f_window)-1))];
            f_window2 = [g, f_window2(1:(length(f_window2)-1))];
        end
             
    end
    
    % Output switching states and its voltage vector. 
    Vi_opt = x_opt; 
    S_opt = states(x_opt,:);
    d_opt = not(S_opt);
    Sopt = [S_opt,d_opt];     

end

== matlab function MPC_MG secondary/Voltage Source Inverter 4/Model Predictive Control  ==
  settings: updateMethod=DISCRETE  sampleTime=Ts
  data: S_opt output; Sopt output size=[1 6]; Vc input; i_filter input; vref input; Vi_opt output; Vdc parameter double size=1; modT parameter size=1; Cfilter parameter size=1; Lfilter parameter size=1
function [S_opt, Sopt, Vi_opt] = MPC(Vc, i_filter,vref,Vdc,modT,Cfilter,Lfilter)

    % In order to call "cont2dis" function
    coder.extrinsic('cont2dis');
    persistent Aq Bq Bdq Vc1 if1 Vc_old if_old x_opt g f_window f_window2 fil fil2

    % Initialize variables and get the parameters of the Discrete model based on Ts
    if isempty(x_opt), x_opt = 1; end
    if isempty(Vc1), Vc1 = 0 + 1j*0; end
    if isempty(Vc_old), Vc_old = 0 + 1j*0; end
    if isempty(if_old), if_old = 0 + 1j*0; end
    if isempty(if1), if1 = 0 + 1j*0; end
    if isempty(f_window), f_window = zeros(1,51); end
    if isempty(f_window2), f_window2 = zeros(1,51); end

    if isempty(Aq) && isempty(Bq) && isempty(Bdq)
        Aq = zeros(2);     Bq = zeros(2,1);     Bdq = zeros(2,1);
        % Call "cont2dis" function
        [Aq, Bq, Bdq] = cont2dis(modT,Lfilter,Cfilter); 
    end
    
    % Intialize the cost function
    g_opt = inf;
    
    % To generate the switching states matrix
    states = [1 0 0;
              0 0 0  
              1 1 0
              0 1 0
              0 1 1
              0 0 1
              1 0 1
              1 1 1];
    a = exp(1j*(2*pi/3));
    %notch filter
    fil = fir1(2,[0.1225 0.1275],'DC-0');
    fil2 = fir1(2,[0.1225 0.1275],'DC-0');
    
    % Read current measurements at sampling instant k
    ifk = i_filter;
    Vck = Vc;
    % Equation of io(k-1) = if(k-1)-(c/Ts)(vc(k)-vc(k-1)).
    io = if_old - (Cfilter/modT)*(Vck - Vc_old); 
    
    % Store the measured current for the next iteration
    if_old = ifk;
    Vc_old = Vck;
    % FOR loop to find the best switch in the next instant and its corresponding V(i)
    for k = 1:8
        s = states(k,:);
        sw = (2/3)*(s(1)+a*s(2)+a^2*s(3));
        Vi = Vdc*sw;

        % Output Voltage Prediction at instant k+1
        if1 = Aq(1,1)*ifk + Aq(1,2)*Vck + Bq(1)*Vi + Bdq(1)*io; 
        Vc1 = Aq(2,1)*ifk + Aq(2,2)*Vck + Bq(2)*Vi + Bdq(2)*io; 
        Nc = sum(abs(states(k,:)-states(x_opt,:)))^2;    
        gf = filter(fil, 1, f_window);
        gf2 = filter(fil2, 1, f_window2);
        g1 = (real(if1)-real(io)+Cfilter*2*pi*50*imag(vref))^2 + (imag(if1)-imag(io)+Cfilter*2*pi*50*real(vref))^2;
        g = (real(vref)-real(Vc1))^2+(imag(vref)-imag(Vc1))^2 + 0.1*g1 + 3*Nc + 3*gf(1) + 3*gf2(1);
        if (g < g_opt)
            x_opt = k;
            g_opt = g;
            f_window = [sqrt((real(vref)-real(Vc1))^2+(imag(vref)-imag(Vc1))^2), f_window(1:(length(f_window)-1))];
            f_window2 = [g, f_window2(1:(length(f_window2)-1))];
        end
             
    end
    
    % Output switching states and its voltage vector. 
    Vi_opt = x_opt; 
    S_opt = states(x_opt,:);
    d_opt = not(S_opt);
    Sopt = [S_opt,d_opt];     

end
